simulink model "SimpleModel1D"  (R2015a)
settings: Solver=ode3  StartTime=0.0  StopTime=tend  FixedStep=1e-3  MaxStep=0.1  RelTol=1e-3
values from neighbouring files (symbols this model uses):
  phi = -param_bar(2)/param_bar(1)    [test2D_data.m]    (also in test_tims_lambda_idea.m = [-param_bar(3)/param_bar(1), -param_bar(2)/param_bar(1) ])
settings Model: CovSFcnEnable=off  Creator=pjseiler  LastModifiedBy=MRDLAB
settings DataIOCC: SignalLoggingSaveFormat=ModelDataLogs
settings OptimizationCC: ExpressionDepthLimit=2147483647
settings DebuggingCC: UnderspecifiedInitializationDetection=Classic  MergeDetectMultiDrivingBlocksExec=none  SolverPrmCheckMsg=warning  MultiTaskDSMMsg=warning  MultiTaskCondExecSysMsg=none  FcnCallInpInsideContextMsg=EnableAllAsWarning  StateNameClashWarn=warning
settings GRTTargetCC: CombineOutputUpdateFcns=off  GRTInterface=on

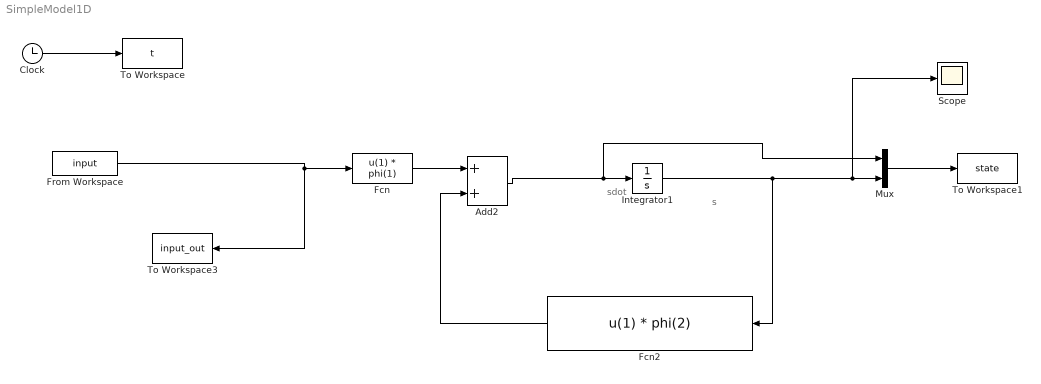
== system SimpleModel1D ==
  note: sdot
  note: s
  Add2 : Sum
  Clock : Clock
  Fcn : Fcn  Expr=u(1) * phi(1)
  Fcn2 : Fcn  Expr=u(1) * phi(2)
  From Workspace : FromWorkspace  VariableName=input  SampleTime=0
  Integrator1 : Integrator
  Mux : Mux  Inputs=2
  Scope : Scope
  To Workspace : ToWorkspace  VariableName=t  SampleTime=-1
  To Workspace1 : ToWorkspace  VariableName=state  SaveFormat=Timeseries  SampleTime=-1
  To Workspace3 : ToWorkspace  VariableName=input_out  SaveFormat=Timeseries  SampleTime=-1
  wires:
  Clock/1 -> To Workspace/1
  Add2/1 -> Mux/1, Integrator1/1
  Integrator1/1 -> Fcn2/1, Mux/2, Scope/1
  Fcn2/1 -> Add2/2
  Mux/1 -> To Workspace1/1
  From Workspace/1 -> Fcn/1, To Workspace3/1
  Fcn/1 -> Add2/1
